simulink model "ComplexPhaseDetector"  (R2016a)
settings: Solver=VariableStepAuto  StartTime=0.0  StopTime=.01  RelTol=1e-6
InitFcn:
  | Bits = 4
  | Ts=3/280e6
  | dBRange=11
  | Br= 1/(10*Ts)
  | EbNo=50
  | FreqOffset=25000
undefined symbols (not defined in the file or in its folder): designMultirateFIR, DiscIntNeverNeededParam
libraries: xbsIndex_r4 x372, dspsigops x5, dspmlti4 x2, commchan3 x2, commdigbbndpm3 x2, simulink x2, dspfdesign x2, commrandsrc3 x2, commanabbnd3 x1
(part 1 of 5)
settings Model: Creator=frank.ziegler  LastModifiedBy=frank

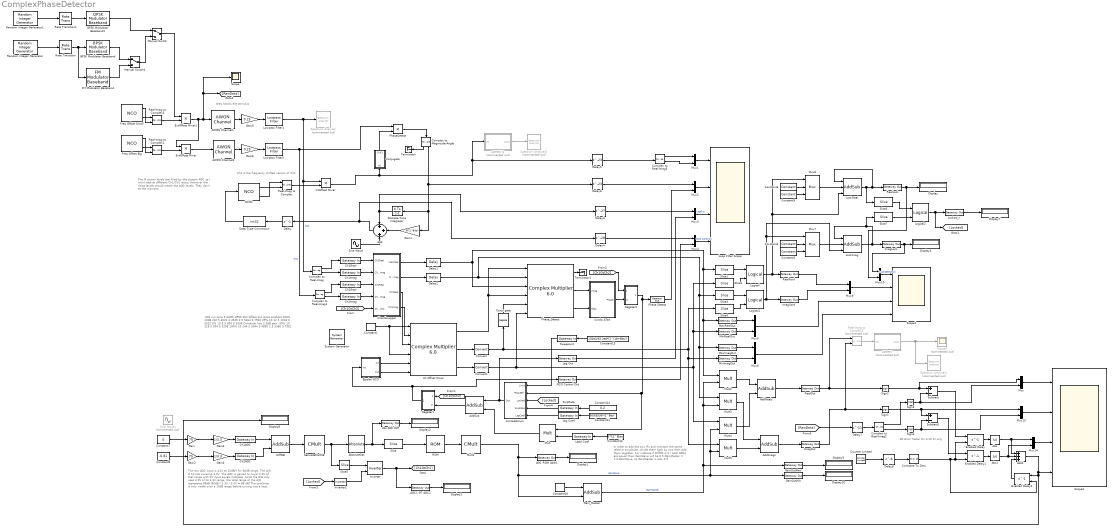
== system ComplexPhaseDetector ==
  note: Bit Error Tester for 1/10 Fs only
  note: .001 run time 9.33Mb QPSK 0Hz Offset but loops enabled
      | 100%	10dB	232
      | 		5		3022
      | 		3		4945
      | 		2.5		5464
      | 		0		7920
      |
      | 39%	10		12
      | 		5		1018
      | 		0		5332
      |
      | 0%		10		8
      | 		5		856
      | 		0		5338	Combiner has 2.5dB gain
      |
      | -39%	10		118
      | 		5		994
      | 		0		5298
      |
      | 100%	10		244
      | 		5		3044
      | 		3		4890
      | 		2.5		5386
      | 		0		7962
  note: The IF power levels are fixed by the system AGC so I won't test at different Ch1/Ch2 ratios.
      | However the noise levels should match the AGC levels. They don't at the moment.
  note: Ch2 is the frequency shifted version of Ch1.
  note: In order to add the two IFs and maintain the same relative amplitude, divide them both by two then add them together.
      | For instance if DiffDb is 0 ( both AGCs are equal) then GainSlave will be 0.5.GainMaster = 1.0-GainSlave, so GainMaster is also 0.5
  note: The raw AGC input is ±2V at 20dB/V for 80dB range.
      |
      | The A/D is 12 bits covering 3.3V. The AGC is gained to cover 3.0V of that range with 0V input equals midscale. Since the A/D only uses 3.0V of its 3.3V range, the total range of the A/D represents 88dB (80dB * 3.3V / 3.0V = 88 dB)
      |
      | The combiner is only viable over a 10dB range before turning into a best source selector. If we only use an eighth of the full range gives us 11dB.
  note: Grey blocks are stimulus
  " Freq Offset Big" : dspsigops/NCO  AccIncSrc=Specify via dialog  AccInc=floor(FreqOffset*Ts*(2^(18+Bits)))  PhaseOffsetSrc=Specify via dialog  PhaseOffset=0  AccumWL=18+Bits  HasDither=off  DitherWL=4  PNgeneratorLength=19  HasPhaseQuantizer=off  TableDepth=12  HasOutputPhaseError=off  Formula=Sine and cosine  DataType=double  OutputWL=16  OutputFL=14  CompMethod=Table lookup (no interpolation)  SampleTime=Ts  SamplesPerFrame=1  OutputFrames=off
  " Freq Offset Small" : dspsigops/NCO  AccIncSrc=Specify via dialog  AccInc=floor(FreqOffset*0.01*Ts*(2^(18+Bits)))  PhaseOffsetSrc=Specify via dialog  PhaseOffset=650000  AccumWL=18+Bits  HasDither=off  DitherWL=4  PNgeneratorLength=19  HasPhaseQuantizer=off  TableDepth=12  HasOutputPhaseError=off  Formula=Sine and cosine  DataType=double  OutputWL=16  OutputFL=14  CompMethod=Table lookup (no interpolation)  SampleTime=Ts  SamplesPerFrame=1  OutputFrames=off
  " System Generator" : xbsIndex_r4/ System Generator  Tag=genX  xilinxfamily=kintex7  part=xc7k325t  speed=-2  package=fbg676  synthesis_tool=Vivado  clock_wrapper=Clock Enables  directory=./netlist  proj_type=Vivado  Synth_file=Vivado Synthesis Defaults  Impl_file=Vivado Implementation Defaults  testbench=off  simulink_period=Ts  sysclk_period=10  dcm_input_clock_period=10  incr_netlist=off  trim_vbits=Everywhere in SubSystem  dbl_ovrd=According to Block Masks  core_generation=According to Block Masks  run_coregen=off  deprecated_control=off  eval_field=0  block_type=sysgen
  AD9957 : Subsystem  Commented=on
  AD9957-2 : Subsystem  Commented=on
  AGC ROM Addr1 : xbsIndex_r4/Gateway Out  inherit_from_input=off  hdl_port=off  rows=1  columns=1  UseAsDAC=off  DACChannel='1'  interface=None  automatic_assignment=on  address_offset=hex2dec('00')  intf_name=''  intf_description=''  timing_constraint=None  locs_specified=off  LOCs={}  io_standard={}  block_type=gatewayout
  AGC1 GT AGC2 : xbsIndex_r4/Gateway Out  inherit_from_input=off  hdl_port=on  rows=1  columns=1  UseAsDAC=off  DACChannel='1'  interface=None  automatic_assignment=on  address_offset=hex2dec('00')  intf_name=''  intf_description=''  timing_constraint=None  locs_specified=off  LOCs={}  io_standard={}  block_type=gatewayout
  AWGN Channel1 : commchan3/AWGN Channel  InputProcessing=Columns as channels (frame based)  seed=67  noiseMode="Signal to noise ratio  (Eb/No)"  EbNodB=EbNo  EsNodB=10  SNRdB=10  bitsPerSym=2  Ps=0.707  Tsym=1/Br  variance=1
  AWGN Channel2 : commchan3/AWGN Channel  InputProcessing=Columns as channels (frame based)  seed=76  noiseMode="Signal to noise ratio  (Eb/No)"  EbNodB=EbNo  EsNodB=10  SNRdB=10  bitsPerSym=2  Ps=0.707  Tsym=1/Br  variance=1
  Abs : Abs
  Abs AGC Diff : xbsIndex_r4/Gateway Out  inherit_from_input=off  hdl_port=on  rows=1  columns=1  UseAsDAC=off  DACChannel='1'  interface=None  automatic_assignment=on  address_offset=hex2dec('00')  intf_name=''  intf_description=''  timing_constraint=None  locs_specified=off  LOCs={}  io_standard={}  block_type=gatewayout
  Abs1 : Abs
  AbsoluteSat : xbsIndex_r4/Absolute  precision=User Defined  arith_type=Unsigned  n_bits=11  bin_pt=11  quantization=Truncate  overflow=Saturate  en=off  latency=1  dbl_ovrd=off  block_type=abs
  Add : Sum  Inputs=+++  OutDataTypeStr=Inherit: Same as first input
  Add1 : Sum  Inputs=+++  AccumDataTypeStr=double  OutDataTypeStr=Inherit: Same as accumulator
  AddImags : xbsIndex_r4/AddSub  mode=Addition  use_carryin=off  use_carryout=off  en=off  latency=1  precision=User Defined  arith_type="Signed  (2's comp)"  n_bits=18  bin_pt=17  quantization="Round  (unbiased: +/- Inf)"  overflow=Saturate  use_behavioral_HDL=off  hw_selection=Fabric  pipelined=off  dbl_ovrd=off  block_type=addsub
  AddReals : xbsIndex_r4/AddSub  mode=Addition  use_carryin=off  use_carryout=off  en=off  latency=1  precision=User Defined  arith_type="Signed  (2's comp)"  n_bits=18  bin_pt=17  quantization="Round  (unbiased: +/- Inf)"  overflow=Saturate  use_behavioral_HDL=off  hw_selection=Fabric  pipelined=off  dbl_ovrd=off  block_type=addsub
  AddSub : xbsIndex_r4/AddSub  mode=Addition  use_carryin=off  use_carryout=off  en=off  latency=1  precision=User Defined  arith_type="Signed  (2's comp)"  n_bits=18+Bits  bin_pt=0  quantization=Truncate  overflow=Wrap  use_behavioral_HDL=off  hw_selection=Fabric  pipelined=off  dbl_ovrd=off  block_type=addsub
  BPSK Modulator Baseband : commdigbbndpm3/BPSK Modulator Baseband  Ph=0  outDtype=double  outWordLen=16  outUDDataType=sfix(16)  outFracLenMode=Best precision  outFracLen=15  outDataTypeStr=double  outLastDataTypeStr=double
  Bipolar NCO : Subsystem
  Ch1AGC : xbsIndex_r4/Gateway In  gui_display_data_type=Fixed-point  arith_type="Signed  (2's comp)"  n_bits=12  bin_pt=11  preci_type=Single  exp_width=8  frac_width=24  rows=1  columns=1  quantization="Round  (unbiased: +/- Inf)"  overflow=Saturate  period=Ts  UseAsADC=off  ADCChannel='1'  interface=None  automatic_assignment=on  address_offset=hex2dec('00')  intf_name=''  intf_description=''  default_value=0  timing_constraint=None  locs_specified=off  LOCs={}  io_standard={}  inherit_from_input=off  hdl_port=on  dbl_ovrd=off  block_type=gatewayin
  Ch1Imag : xbsIndex_r4/Gateway In  gui_display_data_type=Fixed-point  arith_type="Signed  (2's comp)"  n_bits=18  bin_pt=17  preci_type=Single  exp_width=8  frac_width=24  rows=1  columns=1  quantization="Round  (unbiased: +/- Inf)"  overflow=Saturate  period=Ts  UseAsADC=off  ADCChannel='1'  interface=None  automatic_assignment=on  address_offset=hex2dec('00')  intf_name=''  intf_description=''  default_value=0  timing_constraint=None  locs_specified=off  LOCs={}  io_standard={}  inherit_from_input=off  hdl_port=on  dbl_ovrd=off  block_type=gatewayin
  Ch1Real : xbsIndex_r4/Gateway In  gui_display_data_type=Fixed-point  arith_type="Signed  (2's comp)"  n_bits=18  bin_pt=17  preci_type=Single  exp_width=8  frac_width=24  rows=1  columns=1  quantization="Round  (unbiased: +/- Inf)"  overflow=Saturate  period=Ts  UseAsADC=off  ADCChannel='1'  interface=None  automatic_assignment=on  address_offset=hex2dec('00')  intf_name=''  intf_description=''  default_value=0  timing_constraint=None  locs_specified=off  LOCs={}  io_standard={}  inherit_from_input=off  hdl_port=on  dbl_ovrd=off  block_type=gatewayin
  Ch2AGC : xbsIndex_r4/Gateway In  gui_display_data_type=Fixed-point  arith_type="Signed  (2's comp)"  n_bits=12  bin_pt=11  preci_type=Single  exp_width=8  frac_width=24  rows=1  columns=1  quantization="Round  (unbiased: +/- Inf)"  overflow=Saturate  period=Ts  UseAsADC=off  ADCChannel='1'  interface=None  automatic_assignment=on  address_offset=hex2dec('00')  intf_name=''  intf_description=''  default_value=0  timing_constraint=None  locs_specified=off  LOCs={}  io_standard={}  inherit_from_input=off  hdl_port=on  dbl_ovrd=off  block_type=gatewayin
  Ch2Imag : xbsIndex_r4/Gateway In  gui_display_data_type=Fixed-point  arith_type="Signed  (2's comp)"  n_bits=18  bin_pt=17  preci_type=Single  exp_width=8  frac_width=24  rows=1  columns=1  quantization="Round  (unbiased: +/- Inf)"  overflow=Saturate  period=Ts  UseAsADC=off  ADCChannel='1'  interface=None  automatic_assignment=on  address_offset=hex2dec('00')  intf_name=''  intf_description=''  default_value=0  timing_constraint=None  locs_specified=off  LOCs={}  io_standard={}  inherit_from_input=off  hdl_port=on  dbl_ovrd=off  block_type=gatewayin
  Ch2Real : xbsIndex_r4/Gateway In  gui_display_data_type=Fixed-point  arith_type="Signed  (2's comp)"  n_bits=18  bin_pt=17  preci_type=Single  exp_width=8  frac_width=24  rows=1  columns=1  quantization="Round  (unbiased: +/- Inf)"  overflow=Saturate  period=Ts  UseAsADC=off  ADCChannel='1'  interface=None  automatic_assignment=on  address_offset=hex2dec('00')  intf_name=''  intf_description=''  default_value=0  timing_constraint=None  locs_specified=off  LOCs={}  io_standard={}  inherit_from_input=off  hdl_port=on  dbl_ovrd=off  block_type=gatewayin
  ChanSwapper : Subsystem
  Compare To Zero : simulink/Logic and Bit Operations/Compare To Zero  relop===  OutDataTypeStr=boolean
  Complex to Magnitude-Angle : ComplexToMagnitudeAngle
  Complex to Real-Imag{,1..2,5} (4 alike) : ComplexToRealImag
  Conju gate : xbsIndex_r4/Negate  precision=User Defined  arith_type="Signed  (2's comp)"  n_bits=18  bin_pt=17  quantization=Truncate  overflow=Saturate  en=off  latency=0  dbl_ovrd=off  block_type=negate
  Conjugate : Subsystem
  Constant1 : xbsIndex_r4/Constant  const=1  gui_display_data_type=Boolean  arith_type=Boolean  n_bits=16  bin_pt=14  preci_type=Single  exp_width=8  frac_width=24  explicit_period=on  period=Ts  equ=P=C  opselect=C  inp2=PCIN>>17  opr=+  inp1=P  carry=CIN  dbl_ovrd=off  block_type=constant
  Constant10 : xbsIndex_r4/Constant  const=1.0  gui_display_data_type=Fixed-point  arith_type=Unsigned  n_bits=18  bin_pt=18  preci_type=Single  exp_width=8  frac_width=24  explicit_period=on  period=Ts  equ=P=C  opselect=C  inp2=PCIN>>17  opr=+  inp1=P  carry=CIN  dbl_ovrd=off  block_type=constant
  Constant11 : Constant  Value=50/65536*(2^Bits)  OutDataTypeStr=double
  Constant12 : Constant  Value=5*(2^Bits)  OutDataTypeStr=double
  Constant13 : Constant  Value=130e3/93.3e6*(2^(18+Bits))  OutDataTypeStr=double
  Constant14 : Constant  Value=0.2  OutDataTypeStr=double
  Constant4 : xbsIndex_r4/Constant  const=1  gui_display_data_type=Fixed-point  arith_type=Unsigned  n_bits=8  bin_pt=0  preci_type=Single  exp_width=8  frac_width=24  explicit_period=off  period=1  equ=P=C  opselect=C  inp2=PCIN>>17  opr=+  inp1=P  carry=CIN  dbl_ovrd=off  block_type=constant
  Constant5 : xbsIndex_r4/Constant  const=2  gui_display_data_type=Fixed-point  arith_type=Unsigned  n_bits=8  bin_pt=0  preci_type=Single  exp_width=8  frac_width=24  explicit_period=off  period=1  equ=P=C  opselect=C  inp2=PCIN>>17  opr=+  inp1=P  carry=CIN  dbl_ovrd=off  block_type=constant
  Constant6 : xbsIndex_r4/Constant  const=1  gui_display_data_type=Fixed-point  arith_type=Unsigned  n_bits=8  bin_pt=0  preci_type=Single  exp_width=8  frac_width=24  explicit_period=off  period=1  equ=P=C  opselect=C  inp2=PCIN>>17  opr=+  inp1=P  carry=CIN  dbl_ovrd=off  block_type=constant
  Constant7 : Constant  Value=0  OutDataTypeStr=double
  Constant8 : Constant  Value=-0.81  OutDataTypeStr=double
  Constant9 : xbsIndex_r4/Constant  const=2  gui_display_data_type=Fixed-point  arith_type=Unsigned  n_bits=8  bin_pt=0  preci_type=Single  exp_width=8  frac_width=24  explicit_period=off  period=1  equ=P=C  opselect=C  inp2=PCIN>>17  opr=+  inp1=P  carry=CIN  dbl_ovrd=off  block_type=constant
  Convert : xbsIndex_r4/Convert  gui_display_data_type=Fixed-point  arith_type="Signed  (2's comp)"  n_bits=18  bin_pt=17  float_type=Single  exp_bits=8  fraction_bits=24  quantization=Truncate  overflow=Saturate  en=off  latency=1  pipeline=off  dbl_ovrd=off  block_type=convert
  Convert1 : xbsIndex_r4/Convert  gui_display_data_type=Fixed-point  arith_type="Signed  (2's comp)"  n_bits=18  bin_pt=17  float_type=Single  exp_bits=8  fraction_bits=24  quantization=Truncate  overflow=Saturate  en=off  latency=1  pipeline=off  dbl_ovrd=off  block_type=convert
  Cordic ATan : Subsystem
  Counter Limited : simulink/Sources/Counter Limited  uplimit=9  tsamp=-1
  Data Type Conversion : DataTypeConversion  OutDataTypeStr=int32  SaturateOnIntegerOverflow=on
  Delay : Delay  DelayLength=1
  Delay1 : xbsIndex_r4/Delay  rst=off  infoeditControl=Selection of Reset will increase slice count due to use of real FFs and instead of SRLs  en=off  latency=4  reg_retiming=off  dbl_ovrd=off  block_type=delay
  Delay2 : xbsIndex_r4/Delay  rst=off  infoeditControl=Selection of Reset will increase slice count due to use of real FFs and instead of SRLs  en=off  latency=4  reg_retiming=off  dbl_ovrd=off  block_type=delay
  Delay3 : Delay  DelayLength=27
  Delay4 : Delay  DelayLength=28
  Delay5 : Delay  DelayLength=23
  Delay6 : Delay  DelayLength=23
  Delay7 : Delay  DelayLength=11
  Delay8 : Delay  DelayLength=6
  DiffDB : xbsIndex_r4/AddSub  mode=Subtraction  use_carryin=off  use_carryout=off  en=off  latency=1  precision=User Defined  arith_type="Signed  (2's comp)"  n_bits=12  bin_pt=11  quantization=Truncate  overflow=Saturate  use_behavioral_HDL=off  hw_selection=Fabric  pipelined=off  dbl_ovrd=off  block_type=addsub
  Discrete-Time Integrator : DiscreteIntegrator  gainval=(2^Bits)*50/65536/Ts  InitialConditionSetting=State (most efficient)  SampleTime=Ts  ICPrevOutput=DiscIntNeverNeededParam  ICPrevScaledInput=DiscIntNeverNeededParam
  Display{,1..4,7..10} (9 alike) : Display
  Enabled Delay : Delay  DelayLength=1  ShowEnablePort=on
      settings: InputPortMap=u0,e6
  Enabled Delay1 : Delay  DelayLength=1  ShowEnablePort=on
      settings: InputPortMap=u0,e6
  Enabled Delay2 : Delay  DelayLength=1  ShowEnablePort=on
      settings: InputPortMap=u0,e6
  ExtOffset Mixer : Product
  ExtOffset Mixer1 : Product
  FM Modulator Baseband : commanabbnd3/FM Modulator Baseband  FrequencyDeviation=100000  SimulateUsing=Code generation
  Gain : Gain  Gain=.75
  Gain1 : Gain  Gain=5*(2^Bits)
  Gain2 : Gain  Gain=.75
  Gain3 : Gain  Gain=1/3.3
  Gain4 : Gain  Gain=1/3.3
  Gain5 : Gain  Gain=0.25
  Gain6 : Gain  Gain=0.25
  GainOutMax : xbsIndex_r4/Gateway Out  inherit_from_input=off  hdl_port=on  rows=1  columns=1  UseAsDAC=off  DACChannel='1'  interface=None  automatic_assignment=on  address_offset=hex2dec('00')  intf_name=''  intf_description=''  timing_constraint=None  locs_specified=off  LOCs={}  io_standard={}  block_type=gatewayout
  GainOutMin : xbsIndex_r4/Gateway Out  inherit_from_input=off  hdl_port=on  rows=1  columns=1  UseAsDAC=off  DACChannel='1'  interface=None  automatic_assignment=on  address_offset=hex2dec('00')  intf_name=''  intf_description=''  timing_constraint=None  locs_specified=off  LOCs={}  io_standard={}  block_type=gatewayout
  Gain_Master : xbsIndex_r4/AddSub  mode=Subtraction  use_carryin=off  use_carryout=off  en=off  latency=0  precision=User Defined  arith_type=Unsigned  n_bits=18  bin_pt=18  quantization=Truncate  overflow=Wrap  use_behavioral_HDL=off  hw_selection=Fabric  pipelined=off  dbl_ovrd=off  block_type=addsub
  ImagLock : xbsIndex_r4/Gateway Out  inherit_from_input=off  hdl_port=on  rows=1  columns=1  UseAsDAC=off  DACChannel='1'  interface=None  automatic_assignment=on  address_offset=hex2dec('00')  intf_name=''  intf_description=''  timing_constraint=None  locs_specified=off  LOCs={}  io_standard={}  block_type=gatewayout
  ImagOut : xbsIndex_r4/Gateway Out  inherit_from_input=off  hdl_port=on  rows=1  columns=1  UseAsDAC=off  DACChannel='1'  interface=None  automatic_assignment=on  address_offset=hex2dec('00')  intf_name=''  intf_description=''  timing_constraint=None  locs_specified=off  LOCs={}  io_standard={}  block_type=gatewayout
  ImagXord : xbsIndex_r4/Gateway Out  inherit_from_input=off  hdl_port=on  rows=1  columns=1  UseAsDAC=off  DACChannel='1'  interface=None  automatic_assignment=on  address_offset=hex2dec('00')  intf_name=''  intf_description=''  timing_constraint=None  locs_specified=off  LOCs={}  io_standard={}  block_type=gatewayout
  Int Offset Mixer : xbsIndex_r4/Complex Multiplier 6.0   hasatlast=off  hasatuser=off  atuserwidth=1  hasbtlast=off  hasbtuser=off  btuserwidth=1  multtype=Use_Mults  optimizegoal=Resources  flowcontrol=NonBlocking  outputwidth=20  roundmode=Truncate  hasctrltlast=off  hasctrltuser=off  ctrltuserwidth=1  outtlastbehv=Null  latencyconfig=Manual  minimumlatency=3  aclken=off  aresetn=off  trim_axipin_name=on  simulation_type=hybrid_sim  simulation_model=sysgen:cmpy_v6_0  data_path_portlist={ 's_axis_a_tdata_real', 's_axis_a_tdata_imag', 's_axis_b_tdata_real', 's_axis_b_tdata_imag', 's_axis_ctrl_tdata_rounding_bit', 'm_axis_dout_tdata_real', 'm_axis_dout_tdata_imag' }  aportwidth=63  bportwidth=63  ip_name=Complex Multiplier  ip_version=6.0  dsptool_ready=true  ipcore_usecache=true  ipcore_useipmodelcache=true  ipcore_verbose=false  ipcore_latency_parameter='minimumlatency'  wrapper_available=true  port_translation_map={ 'aclken' => 'en', 'aresetn' => 'rst'}  block_type=cmpy_v6_0
  IntOffset Mixer : Product
  Inverter : xbsIndex_r4/Inverter  en=on  latency=01  dbl_ovrd=off  block_type=inv
  Inverter2 : xbsIndex_r4/Inverter  en=off  latency=0  dbl_ovrd=off  block_type=inv
  Lag Coef : xbsIndex_r4/Gateway In  gui_display_data_type=Fixed-point  arith_type="Signed  (2's comp)"  n_bits=18  bin_pt=17  preci_type=Single  exp_width=8  frac_width=24  rows=1  columns=1  quantization="Round  (unbiased: +/- Inf)"  overflow=Wrap  period=Ts  UseAsADC=off  ADCChannel='1'  interface=None  automatic_assignment=on  address_offset=hex2dec('00')  intf_name='axi4'  intf_description='Lead Coefficient'  default_value=5*Ts  timing_constraint=None  locs_specified=off  LOCs={}  io_standard={}  inherit_from_input=off  hdl_port=on  dbl_ovrd=off  block_type=gatewayin
  Lag Out : xbsIndex_r4/Gateway Out  inherit_from_input=off  hdl_port=on  rows=1  columns=1  UseAsDAC=off  DACChannel='1'  interface=None  automatic_assignment=on  address_offset=hex2dec('00')  intf_name=''  intf_description=''  timing_constraint=None  locs_specified=off  LOCs={}  io_standard={}  block_type=gatewayout
  Lead Coef : xbsIndex_r4/Gateway In  gui_display_data_type=Fixed-point  arith_type="Signed  (2's comp)"  n_bits=18  bin_pt=9  preci_type=Single  exp_width=8  frac_width=24  rows=1  columns=1  quantization="Round  (unbiased: +/- Inf)"  overflow=Wrap  period=Ts  UseAsADC=off  ADCChannel='1'  interface=None  automatic_assignment=on  address_offset=hex2dec('00')  intf_name='axi4'  intf_description='Lead Coefficient'  default_value=10  timing_constraint=None  locs_specified=off  LOCs={}  io_standard={}  inherit_from_input=off  hdl_port=on  dbl_ovrd=off  block_type=gatewayin
  LimitedAccum : Subsystem
  LockImag : xbsIndex_r4/AddSub  mode=Addition or Subtraction  use_carryin=off  use_carryout=off  en=off  latency=1  precision=User Defined  arith_type=Unsigned  n_bits=13  bin_pt=0  quantization=Truncate  overflow=Saturate  use_behavioral_HDL=off  hw_selection=Fabric  pipelined=off  dbl_ovrd=off  block_type=addsub
  LockReal : xbsIndex_r4/AddSub  mode=Addition or Subtraction  use_carryin=off  use_carryout=off  en=off  latency=1  precision=User Defined  arith_type=Unsigned  n_bits=13  bin_pt=0  quantization=Truncate  overflow=Saturate  use_behavioral_HDL=off  hw_selection=Fabric  pipelined=off  dbl_ovrd=off  block_type=addsub
  Locked_n : xbsIndex_r4/Gateway Out  inherit_from_input=off  hdl_port=on  rows=1  columns=1  UseAsDAC=off  DACChannel='1'  interface=None  automatic_assignment=on  address_offset=hex2dec('00')  intf_name=''  intf_description=''  timing_constraint=None  locs_specified=off  LOCs={}  io_standard={}  block_type=gatewayout
  Logical : xbsIndex_r4/Logical  logical_function=XOR  inputs=2  en=off  latency=1  precision=Full  arith_type=Unsigned  n_bits=16  bin_pt=0  align_bp=on  dbl_ovrd=off  block_type=logical
  Logical1 : xbsIndex_r4/Logical  logical_function=XOR  inputs=2  en=off  latency=1  precision=Full  arith_type=Unsigned  n_bits=16  bin_pt=0  align_bp=on  dbl_ovrd=off  block_type=logical
  Logical2 : xbsIndex_r4/Logical  logical_function=OR  inputs=2  en=off  latency=1  precision=Full  arith_type=Unsigned  n_bits=16  bin_pt=0  align_bp=on  dbl_ovrd=off  block_type=logical
  Loop Filter Scope : Scope  NumInputPorts=4
  Lowpass Filter1 : dspfdesign/Lowpass Filter  FilterType=FIR  DesignForMinimumOrder=on  FilterOrder=50  PassbandFrequency=Br/2  StopbandFrequency=46e6  PassbandRipple=0.1  StopbandAttenuation=80  InheritSampleRate=off  SampleRate=1/Ts  roundingMode=Floor  coeffsDataTypeStr=fixdt(1,16)  SimulateUsing=Interpreted execution
  Lowpass Filter2 : dspfdesign/Lowpass Filter  FilterType=FIR  DesignForMinimumOrder=on  FilterOrder=50  PassbandFrequency=Br/2  StopbandFrequency=46e6  PassbandRipple=0.1  StopbandAttenuation=80  InheritSampleRate=off  SampleRate=1/Ts  roundingMode=Floor  coeffsDataTypeStr=fixdt(1,16)  SimulateUsing=Interpreted execution
  Manual Switch : ManualSwitch
  Manual Switch1 : ManualSwitch
  MaxImagOut : xbsIndex_r4/Gateway Out  inherit_from_input=off  hdl_port=on  rows=1  columns=1  UseAsDAC=off  DACChannel='1'  interface=None  automatic_assignment=on  address_offset=hex2dec('00')  intf_name=''  intf_description=''  timing_constraint=None  locs_specified=off  LOCs={}  io_standard={}  block_type=gatewayout
  MaxRealOut : xbsIndex_r4/Gateway Out  inherit_from_input=off  hdl_port=on  rows=1  columns=1  UseAsDAC=off  DACChannel='1'  interface=None  automatic_assignment=on  address_offset=hex2dec('00')  intf_name=''  intf_description=''  timing_constraint=None  locs_specified=off  LOCs={}  io_standard={}  block_type=gatewayout
  MinImagOut : xbsIndex_r4/Gateway Out  inherit_from_input=off  hdl_port=on  rows=1  columns=1  UseAsDAC=off  DACChannel='1'  interface=None  automatic_assignment=on  address_offset=hex2dec('00')  intf_name=''  intf_description=''  timing_constraint=None  locs_specified=off  LOCs={}  io_standard={}  block_type=gatewayout
  MinRealOut : xbsIndex_r4/Gateway Out  inherit_from_input=off  hdl_port=on  rows=1  columns=1  UseAsDAC=off  DACChannel='1'  interface=None  automatic_assignment=on  address_offset=hex2dec('00')  intf_name=''  intf_description=''  timing_constraint=None  locs_specified=off  LOCs={}  io_standard={}  block_type=gatewayout
  Mult : xbsIndex_r4/Mult  precision=User Defined  arith_type="Signed  (2's comp)"  n_bits=18+Bits  bin_pt=9  quantization="Round  (unbiased: +/- Inf)"  overflow=Wrap  en=off  latency=4  use_behavioral_HDL=off  opt=Speed  use_embedded=on  optimum_pipeline=off  pipeline=on  dbl_ovrd=off  use_rpm=on  placement_style=Triangular  block_type=mult
  Mult1 : xbsIndex_r4/CMult  const=0.5  gui_display_data_type=Fixed-point  const_n_bits=4  const_bin_pt=3  float_type=Single  exp_bits=8  fraction_bits=24  en=off  latency=0  precision=User Defined  arith_type=Unsigned  n_bits=18  bin_pt=18  quantization=Truncate  overflow=Wrap  use_behavioral_HDL=off  mem_type=Distributed RAM  pipeline=off  dbl_ovrd=off  block_type=cmult
  Mult{2..5} (4 alike) : xbsIndex_r4/Mult  precision=User Defined  arith_type="Signed  (2's comp)"  n_bits=18  bin_pt=17  quantization="Round  (unbiased: +/- Inf)"  overflow=Wrap  en=off  latency=3  use_behavioral_HDL=off  opt=Speed  use_embedded=on  optimum_pipeline=off  pipeline=on  dbl_ovrd=off  use_rpm=on  placement_style=Triangular  block_type=mult
  Mux{,1..6,9..10,13..14} (11 alike) : Mux  Inputs=2
  Mux7 : xbsIndex_r4/Mux  inputs=2  en=off  latency=0  precision=Full  arith_type=Unsigned  n_bits=16  bin_pt=14  quantization=Truncate  overflow=Wrap  dbl_ovrd=off  block_type=mux
  Mux8 : xbsIndex_r4/Mux  inputs=2  en=off  latency=0  precision=Full  arith_type=Unsigned  n_bits=16  bin_pt=14  quantization=Truncate  overflow=Wrap  dbl_ovrd=off  block_type=mux
  NCO Control Out : xbsIndex_r4/Gateway Out  inherit_from_input=off  hdl_port=on  rows=1  columns=1  UseAsDAC=off  DACChannel='1'  interface=None  automatic_assignment=on  address_offset=hex2dec('00')  intf_name=''  intf_description=''  timing_constraint=None  locs_specified=off  LOCs={}  io_standard={}  block_type=gatewayout
  NCO1 : dspsigops/NCO  AccIncSrc=Input port  AccInc=100  PhaseOffsetSrc=Specify via dialog  PhaseOffset=0  AccumWL=18+Bits  HasDither=off  DitherWL=4  PNgeneratorLength=19  HasPhaseQuantizer=off  TableDepth=12  HasOutputPhaseError=off  Formula=Sine and cosine  DataType=double  OutputWL=16  OutputFL=14  CompMethod=Table lookup (no interpolation)  SampleTime=Ts  SamplesPerFrame=1  OutputFrames=off
  Negater1 : Subsystem
  Negater2 : Subsystem
  Phase Detect : xbsIndex_r4/Gateway Out  inherit_from_input=off  hdl_port=on  rows=1  columns=1  UseAsDAC=off  DACChannel='1'  interface=None  automatic_assignment=on  address_offset=hex2dec('00')  intf_name=''  intf_description=''  timing_constraint=None  locs_specified=off  LOCs={}  io_standard={}  block_type=gatewayout
  PhaseDetect : Product
  Phase_Detect : xbsIndex_r4/Complex Multiplier 6.0   hasatlast=off  hasatuser=off  atuserwidth=1  hasbtlast=off  hasbtuser=off  btuserwidth=1  multtype=Use_Mults  optimizegoal=Resources  flowcontrol=NonBlocking  outputwidth=18  roundmode=Truncate  hasctrltlast=off  hasctrltuser=off  ctrltuserwidth=1  outtlastbehv=Null  latencyconfig=Automatic  minimumlatency=37  aclken=off  aresetn=off  trim_axipin_name=on  simulation_type=hybrid_sim  simulation_model=sysgen:cmpy_v6_0  data_path_portlist={ 's_axis_a_tdata_real', 's_axis_a_tdata_imag', 's_axis_b_tdata_real', 's_axis_b_tdata_imag', 's_axis_ctrl_tdata_rounding_bit', 'm_axis_dout_tdata_real', 'm_axis_dout_tdata_imag' }  aportwidth=63  bportwidth=63  ip_name=Complex Multiplier  ip_version=6.0  dsptool_ready=true  ipcore_usecache=true  ipcore_useipmodelcache=true  ipcore_verbose=false  ipcore_latency_parameter='minimumlatency'  wrapper_available=true  port_translation_map={ 'aclken' => 'en', 'aresetn' => 'rst'}  block_type=cmpy_v6_0
  QPSK Modulator Baseband1 : commdigbbndpm3/QPSK Modulator Baseband  InType=Integer  Enc=Gray  Ph=pi/4  outDtype=double  outWordLen=16  outUDDataType=sfix(16)  outFracLenMode=Best precision  outFracLen=15  outDataTypeStr=double  outLastDataTypeStr=double
  ROM : xbsIndex_r4/ROM  depth=1024  initVector=[10.^((0:1022)*(-(dBRange/20))/1023) 0]  distributed_mem=Block RAM  rst=off  init_reg=0  en=off  latency=1  gui_display_data_type=Fixed-point  arith_type=Unsigned  n_bits=18  bin_pt=18  preci_type=Single  exp_width=8  frac_width=24  optimize=Area  use_rpm=on  dbl_ovrd=off  block_type=sprom
  Random Integer Generator : commrandsrc3/Random Integer Generator  SetSize=2  SeedSource=Auto  Seed=0  SampleTime=1/Br  SamplesPerFrame=1  OutputDataType=double  SimulateUsing=Code generation
  Random Integer Generator1 : commrandsrc3/Random Integer Generator  SetSize=4  SeedSource=Auto  Seed=0  SampleTime=1/Br  SamplesPerFrame=1  OutputDataType=double  SimulateUsing=Code generation
  Rate Transition : RateTransition  OutPortSampleTime=Ts
  Rate Transition1 : RateTransition  OutPortSampleTime=Ts
  Real-Imag to Complex : RealImagToComplex
  Real-Imag to Complex1 : RealImagToComplex
  Real-Imag to Complex2 : RealImagToComplex  Commented=on
  Real-Imag to Complex3 : RealImagToComplex
  RealLock : xbsIndex_r4/Gateway Out  inherit_from_input=off  hdl_port=on  rows=1  columns=1  UseAsDAC=off  DACChannel='1'  interface=None  automatic_assignment=on  address_offset=hex2dec('00')  intf_name=''  intf_description=''  timing_constraint=None  locs_specified=off  LOCs={}  io_standard={}  block_type=gatewayout
  RealOut : xbsIndex_r4/Gateway Out  inherit_from_input=off  hdl_port=on  rows=1  columns=1  UseAsDAC=off  DACChannel='1'  interface=None  automatic_assignment=on  address_offset=hex2dec('00')  intf_name=''  intf_description=''  timing_constraint=None  locs_specified=off  LOCs={}  io_standard={}  block_type=gatewayout
  RealXord : xbsIndex_r4/Gateway Out  inherit_from_input=off  hdl_port=on  rows=1  columns=1  UseAsDAC=off  DACChannel='1'  interface=None  automatic_assignment=on  address_offset=hex2dec('00')  intf_name=''  intf_description=''  timing_constraint=None  locs_specified=off  LOCs={}  io_standard={}  block_type=gatewayout
  SaturateMultX8 : xbsIndex_r4/CMult  const=8  gui_display_data_type=Fixed-point  const_n_bits=4  const_bin_pt=0  float_type=Single  exp_bits=8  fraction_bits=24  en=off  latency=0  precision=User Defined  arith_type="Signed  (2's comp)"  n_bits=18  bin_pt=17  quantization=Truncate  overflow=Saturate  use_behavioral_HDL=off  mem_type=Distributed RAM  pipeline=off  dbl_ovrd=off  block_type=cmult
  Scope : Scope
  Scope1 : Scope  NumInputPorts=4
  Scope3 : Scope  NumInputPorts=4
  Scope5 : Scope  Commented=on
  Sign{1..4} (4 alike) : Signum
  Sine Wave : Sin  Amplitude=0  Frequency=2*2*pi()  SampleTime=Ts
  Sine Wave1 : Sin  Commented=on  Frequency=2000  SampleTime=Ts
  Slice : xbsIndex_r4/Slice  nbits=10  boolean_output=off  mode=Upper Bit Location + Width  bit1=0  base1=MSB of Input  bit0=0  base0=LSB of Input  dbl_ovrd=off  block_type=slice
  Slice{1..7} (7 alike) : xbsIndex_r4/Slice  nbits=1  boolean_output=on  mode=Upper Bit Location + Width  bit1=0  base1=MSB of Input  bit0=0  base0=LSB of Input  dbl_ovrd=off  block_type=slice
  Spectrum Analyzer : SpectrumAnalyzer  Commented=on
  Spectrum Analyzer1 : SpectrumAnalyzer  Commented=on
  Spectrum Analyzer2 : SpectrumAnalyzer  Commented=on
  Subtract : Sum  Inputs=+-
  Subtract1 : Sum  Inputs=+-
  SweepLmt : xbsIndex_r4/Gateway In  gui_display_data_type=Fixed-point  arith_type="Signed  (2's comp)"  n_bits=10+Bits  bin_pt=0  preci_type=Single  exp_width=8  frac_width=24  rows=1  columns=1  quantization="Round  (unbiased: +/- Inf)"  overflow=Wrap  period=Ts  UseAsADC=off  ADCChannel='1'  interface=None  automatic_assignment=on  address_offset=hex2dec('00')  intf_name='axi4'  intf_description='Lead Coefficient'  default_value=5*Ts  timing_constraint=None  locs_specified=off  LOCs={}  io_standard={}  inherit_from_input=off  hdl_port=on  dbl_ovrd=off  block_type=gatewayin
  SwpRate : xbsIndex_r4/Gateway In  gui_display_data_type=Fixed-point  arith_type="Signed  (2's comp)"  n_bits=18  bin_pt=9  preci_type=Single  exp_width=8  frac_width=24  rows=1  columns=1  quantization="Round  (unbiased: +/- Inf)"  overflow=Wrap  period=Ts  UseAsADC=off  ADCChannel='1'  interface=None  automatic_assignment=on  address_offset=hex2dec('00')  intf_name='axi4'  intf_description='Lead Coefficient'  default_value=5*Ts  timing_constraint=None  locs_specified=off  LOCs={}  io_standard={}  inherit_from_input=off  hdl_port=on  dbl_ovrd=off  block_type=gatewayin
  Terminator : Terminator
  Terminator1 : Terminator
  wires:
  Real-Imag to Complex/1 -> IntOffset Mixer/2
  PhaseDetect/1 -> Complex to Magnitude-Angle/1
  Conjugate/1(Out1) -> PhaseDetect/2
  NCO1/2 -> Real-Imag to Complex/1
  NCO1/1 -> Real-Imag to Complex/2
  Discrete-Time Integrator/1 -> Delay3/1, Add/1
  Gain1/1 -> Add/2
  Sine Wave/1 -> Add/3
  ExtOffset Mixer1/1 -> ExtOffset Mixer/1, Scope/1, [RawData], AWGN Channel1/1
  " Freq Offset Big"/1 -> Real-Imag to Complex1/2
  " Freq Offset Big"/2 -> Real-Imag to Complex1/1
  Real-Imag to Complex1/1 -> ExtOffset Mixer/2
  IntOffset Mixer/1 -> AD9957-2/1(In1), Delay5/1, Conjugate/1(In1)
  Complex to Magnitude-Angle/2 -> Delay6/1, Gain1/1, Discrete-Time Integrator/1
  Complex to Real-Imag/1 -> Ch1Real/1
  Complex to Real-Imag/2 -> Ch1Imag/1
  Complex to Real-Imag1/2 -> Ch2Imag/1
  Complex to Real-Imag1/1 -> Ch2Real/1
  Int Offset Mixer/2 -> Convert/1
  Int Offset Mixer/1 -> Phase_Detect/4, Phase_Detect/1
  Conju gate/1 -> Phase_Detect/5
  Complex to Magnitude-Angle/1 -> Terminator/1
  Constant1/1 -> Int Offset Mixer/4, Int Offset Mixer/1
  Mult/1 -> AddSub/2
  Phase Detect/1 -> Mux2/2
  Int Offset Mixer/3 -> Convert1/1
  Lead Coef/1 -> Mult/2
  Lag Coef/1 -> LimitedAccum/5(LagCoef)
  Data Type Conversion/1 -> NCO1/1
  Bipolar NCO/1(sin) -> Int Offset Mixer/5
  Bipolar NCO/2(cos) -> Int Offset Mixer/6
  Phase_Detect/1 -> Terminator1/1
  MaxRealOut/1 -> Mux5/1
  MaxImagOut/1 -> Mux6/1
  MinImagOut/1 -> Mux6/2
  MinRealOut/1 -> Mux5/2
  Convert/1 -> MinImagOut/1, Mult5/1, Slice4/1, Conju gate/1
  Convert1/1 -> Phase_Detect/6, Slice2/1, MinRealOut/1, Mult4/1
  Mux5/1 -> Scope1/3
  Mux6/1 -> Scope1/4
  Mult1/1 -> AGC ROM Addr1/1, Gain_Master/2, GainOutMin/1, Mult4/2, Mult5/2  "GainSlave"
  Ch1AGC/1 -> DiffDB/1
  Ch2AGC/1 -> DiffDB/2
  DiffDB/1 -> SaturateMultX8/1
  Constant8/1 -> Gain2/1
  Gain/1 -> Gain3/1
  Gain2/1 -> Gain4/1
  Gain4/1 -> Ch2AGC/1
  Gain3/1 -> Ch1AGC/1
  AbsoluteSat/1 -> Slice/1, Abs AGC Diff/1
  Abs AGC Diff/1 -> Display2/1
  AGC1 GT AGC2/1 -> Display3/1
  SaturateMultX8/1 -> AbsoluteSat/1, Slice5/1
  Mult2/1 -> AddReals/1
  Mult4/1 -> AddReals/2
  Mult5/1 -> AddImags/2
  Mult3/1 -> AddImags/1
  AddReals/1 -> RealOut/1
  Inverter/1 -> [Ch1GtCh2], AGC1 GT AGC2/1
  Constant10/1 -> Gain_Master/1
  ROM/1 -> Mult1/1
  RealOut/1 -> Sign2/1, Real-Imag to Complex2/1
  ImagOut/1 -> Real-Imag to Complex2/2, Sign1/1
  AddImags/1 -> ImagOut/1
  Constant11/1 -> Lag Coef/1
  Constant12/1 -> Lead Coef/1
  AWGN Channel1/1 -> Gain5/1
  Gain5/1 -> Lowpass Filter1/1
  Phase_Detect/2 -> Cordic ATan/1(Imag)
  Phase_Detect/3 -> Cordic ATan/2(Real)
  AWGN Channel2/1 -> Gain6/1
  Gain6/1 -> Lowpass Filter2/1
  ExtOffset Mixer/1 -> AWGN Channel2/1
  Complex to Real-Imag5/1 -> Mux1/1
  Complex to Real-Imag5/2 -> Mux1/2
  Lag Out/1 -> Mux3/2
  Real-Imag to Complex2/1 -> AD9957/1(In1)
  Rate Transition/1 -> FM Modulator Baseband/1, BPSK Modulator Baseband/1
  Random Integer Generator/1 -> Rate Transition/1
  AD9957/1(Out1) -> Scope5/1, Spectrum Analyzer1/1
  Delay3/1 -> Mux3/1
  Delay5/1 -> Complex to Real-Imag5/1
  Delay6/1 -> Mux2/1
  AD9957-2/1(Out1) -> Spectrum Analyzer2/1
  Slice/1 -> ROM/1
  AGC ROM Addr1/1 -> Display1/1
  Slice1/1 -> Logical/1
  Slice2/1 -> Logical/2
  RealXord/1 -> Mux9/1
  Slice3/1 -> Logical1/1
  Slice4/1 -> Logical1/2
  ImagXord/1 -> Mux9/2
  LockReal/1 -> Slice6/1, LockReal/1, RealLock/1
  RealLock/1 -> Mux10/2, Display/1
  Mux9/1 -> Scope1/2
  Logical1/1 -> LockImag/3, Mux7/1, ImagXord/1
  LockImag/1 -> Slice7/1, LockImag/1, ImagLock/1
  Mux7/1 -> LockImag/2
  ImagLock/1 -> Display4/1, Mux10/1
  Mux10/1 -> Scope1/1  "LockDetectors"
  [Ch1GtCh2] -> ChanSwapper/5(Ch1GtCh2)
  Slice5/1 -> Inverter/1
  Delay/1 -> Data Type Conversion/1
  Mux3/1 -> Loop Filter Scope/3  "LagOut"
  Mux4/1 -> Loop Filter Scope/4  "NCO Controls"
  Delay4/1 -> Mux4/1
  NCO Control Out/1 -> Mux4/2
  Ch1Imag/1 -> ChanSwapper/2(Ch1Imag)
  Ch2Real/1 -> ChanSwapper/3(Ch2Real)
  Ch2Imag/1 -> ChanSwapper/4(Ch2Imag)
  Ch1Real/1 -> ChanSwapper/1(Ch1Real)
  ChanSwapper/4(MinImag) -> Int Offset Mixer/2
  ChanSwapper/3("MinReal ") -> Int Offset Mixer/3
  Lowpass Filter1/1 -> Spectrum Analyzer/1, Complex to Real-Imag/1, IntOffset Mixer/1  "Ch1"
  Lowpass Filter2/1 -> PhaseDetect/1, Complex to Real-Imag1/1  "Ch2"
  Constant4/1 -> Mux7/2
  Constant5/1 -> Mux7/3
  Logical/1 -> Mux8/1, LockReal/3, RealXord/1
  Mux8/1 -> LockReal/2
  Constant6/1 -> Mux8/2
  Constant9/1 -> Mux8/3
  Negater1/1(Out) -> NCO Control Out/1, Bipolar NCO/1(Inc)
  [Ch1GtCh2] -> Negater1/1(Sel)
  AddSub/1 -> Negater1/2(In)
  Cordic ATan/1(Phase) -> Negater2/2(In)
  [Ch1GtCh2] -> Negater2/1(Sel)
  Add/1 -> Delay4/1, Delay/1
  Slice7/1 -> Logical2/2
  Slice6/1 -> Logical2/1
  Logical2/1 -> Locked_n/1, [Locked]
  Locked_n/1 -> Display7/1
  Mux1/1 -> Loop Filter Scope/1
  Mux2/1 -> Loop Filter Scope/2
  [Locked] -> Inverter2/1
  LimitedAccum/1(Out) -> AddSub/1, Lag Out/1
  Negater2/1(Out) -> LimitedAccum/2(PhaseErr), Mult/1, Phase Detect/1
  SweepLmt/1 -> LimitedAccum/1(Limit)
  Constant13/1 -> SweepLmt/1
  ChanSwapper/1(MaxReal) -> Delay1/1
  ChanSwapper/2(MaxImag) -> Delay2/1
  Delay2/1 -> Slice3/1, Mult3/1, MaxImagOut/1, Phase_Detect/2
  Delay1/1 -> Phase_Detect/3, Mult2/1, MaxRealOut/1, Slice1/1
  Constant14/1 -> SwpRate/1
  SwpRate/1 -> LimitedAccum/4(SwpRate)
  [Locked] -> LimitedAccum/3(Locked)
  Gain_Master/1 -> GainOutMax/1, Mult3/2, Mult2/2  "GainMaster"
  Inverter2/1 -> Inverter/2
  Constant7/1 -> Gain/1
  Complex to Real-Imag2/2 -> Sign4/1
  Complex to Real-Imag2/1 -> Sign3/1
  Delay7/1 -> Complex to Real-Imag2/1
  Subtract1/1 -> Enabled Delay1/1
  Subtract/1 -> Enabled Delay/1
  Counter Limited/1 -> Delay8/1
  Enabled Delay/1 -> Abs/1
  Enabled Delay1/1 -> Abs1/1
  Mux/1 -> Scope3/1
  Mux13/1 -> Scope3/2
  Mux14/1 -> Scope3/3
  Sign2/1 -> Mux/1, Subtract/1
  Sign1/1 -> Subtract1/1, Mux13/1
  Sign3/1 -> Mux/2, Subtract/2
  Sign4/1 -> Mux13/2, Subtract1/2
  Delay8/1 -> Compare To Zero/1
  Abs/1 -> Add1/1, Mux14/1
  Abs1/1 -> Add1/2, Mux14/2
  Add1/1 -> Enabled Delay2/1, Display8/1, Scope3/4
  Enabled Delay2/1 -> Add1/3
  Compare To Zero/1 -> Enabled Delay2/2, Enabled Delay1/2, Enabled Delay/2
  GainOutMax/1 -> Display9/1
  GainOutMin/1 -> Display10/1
  [RawData] -> Delay7/1
  Manual Switch/1 -> ExtOffset Mixer1/1
  " Freq Offset Small"/1 -> Real-Imag to Complex3/2
  " Freq Offset Small"/2 -> Real-Imag to Complex3/1
  Real-Imag to Complex3/1 -> ExtOffset Mixer1/2
  Random Integer Generator1/1 -> Rate Transition1/1
  Rate Transition1/1 -> QPSK Modulator Baseband1/1
  QPSK Modulator Baseband1/1 -> Manual Switch/1
  BPSK Modulator Baseband/1 -> Manual Switch1/1
  FM Modulator Baseband/1 -> Manual Switch1/2
  Manual Switch1/1 -> Manual Switch/2

== system ComplexPhaseDetector/AD9957 ==
  In1 : Inport
  Add3 : Sum
  Complex to Real-Imag3 : ComplexToRealImag
  FIR Interpolation : dspmlti4/FIR Interpolation  FilterSource=Auto  h=designMultirateFIR(3,1)  L=8  FilterObject=FINTERP  framing=Allow multirate processing  outputBufInitCond=0  roundingMode=Floor  overflowMode=off  firstCoeffDataTypeStr=Inherit: Same word length as input  firstCoeffMin=[]  firstCoeffMax=[]  firstCoeffLastDataTypeStr=Inherit: Same word length as input  outputDataTypeStr=Inherit: Same as accumulator  outputMin=[]  outputMax=[]  outputLastDataTypeStr=Inherit: Same as accumulator
  NCO : dspsigops/NCO  AccIncSrc=Specify via dialog  AccInc=16384*3/8  PhaseOffsetSrc=Specify via dialog  PhaseOffset=0  AccumWL=16  HasDither=off  DitherWL=4  PNgeneratorLength=19  HasPhaseQuantizer=off  TableDepth=12  HasOutputPhaseError=off  Formula=Sine and cosine  DataType=double  OutputWL=16  OutputFL=14  CompMethod=Table lookup (no interpolation)  SampleTime=Ts/8  SamplesPerFrame=1  OutputFrames=off
  PhaseDetect1 : Product
  PhaseDetect2 : Product
  Out1 : Outport
  wires:
  In1/1 -> FIR Interpolation/1
  NCO/1 -> PhaseDetect2/2
  Complex to Real-Imag3/1 -> PhaseDetect1/1
  PhaseDetect2/1 -> Add3/1
  PhaseDetect1/1 -> Add3/2
  Complex to Real-Imag3/2 -> PhaseDetect2/1
  FIR Interpolation/1 -> Complex to Real-Imag3/1
  NCO/2 -> PhaseDetect1/2
  Add3/1 -> Out1/1

== system ComplexPhaseDetector/AD9957-2 ==
  In1 : Inport
  Add3 : Sum
  Complex to Real-Imag3 : ComplexToRealImag
  FIR Interpolation : dspmlti4/FIR Interpolation  FilterSource=Auto  h=designMultirateFIR(3,1)  L=8  FilterObject=FINTERP  framing=Allow multirate processing  outputBufInitCond=0  roundingMode=Floor  overflowMode=off  firstCoeffDataTypeStr=Inherit: Same word length as input  firstCoeffMin=[]  firstCoeffMax=[]  firstCoeffLastDataTypeStr=Inherit: Same word length as input  outputDataTypeStr=Inherit: Same as accumulator  outputMin=[]  outputMax=[]  outputLastDataTypeStr=Inherit: Same as accumulator
  NCO : dspsigops/NCO  AccIncSrc=Specify via dialog  AccInc=16384*3/8  PhaseOffsetSrc=Specify via dialog  PhaseOffset=0  AccumWL=16  HasDither=off  DitherWL=4  PNgeneratorLength=19  HasPhaseQuantizer=off  TableDepth=12  HasOutputPhaseError=off  Formula=Sine and cosine  DataType=double  OutputWL=16  OutputFL=14  CompMethod=Table lookup (no interpolation)  SampleTime=Ts/8  SamplesPerFrame=1  OutputFrames=off
  PhaseDetect1 : Product
  PhaseDetect2 : Product
  Out1 : Outport
  wires:
  Add3/1 -> Out1/1
  NCO/2 -> PhaseDetect1/2
  FIR Interpolation/1 -> Complex to Real-Imag3/1
  Complex to Real-Imag3/2 -> PhaseDetect2/1
  PhaseDetect1/1 -> Add3/2
  PhaseDetect2/1 -> Add3/1
  Complex to Real-Imag3/1 -> PhaseDetect1/1
  NCO/1 -> PhaseDetect2/2
  In1/1 -> FIR Interpolation/1

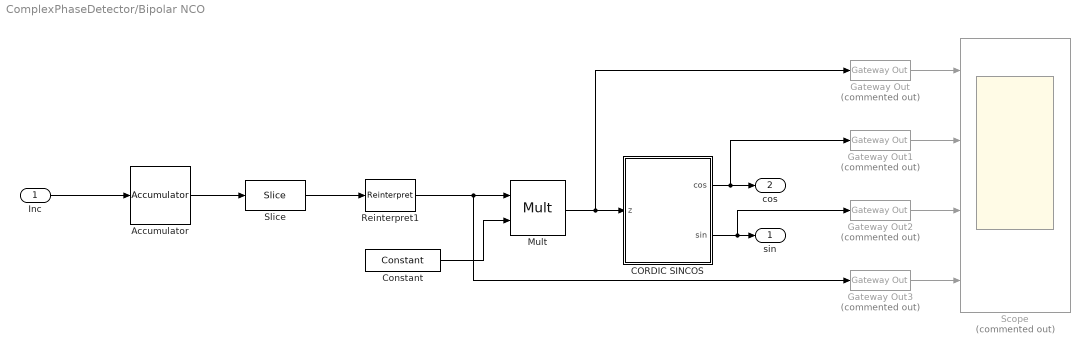
== system ComplexPhaseDetector/Bipolar NCO ==
  Inc : Inport
  Accumulator : xbsIndex_r4/Accumulator  operation=Add  n_bits=18+Bits  overflow=Wrap  scale=1  rst=off  hasbypass=off  infoeditControl=reset for floating point data type must be asserted for a minimum of 2 cycles  en=off  latency=1  msb_inp=100  msb=100  lsb=-100  use_behavioral_HDL=on  implementation=Fabric  dbl_ovrd=off  block_type=accum
  CORDIC SINCOS : Subsystem  mask(Xilinx CORDIC SINCOS){stages=17, pe_nbits=21, pe_binpt=17, pipeline_x=ones(1,17), prev_stages=17, pipeline=[1  1  1  1  1  1  1  1  1  1  1  1  1  1  1  1  1]}
      mask prompts: stages "Number of Processing Elements (integer value starting from 1)"; pe_nbits "Input Data Width"; pe_binpt "Input Binary Point Position"; pipeline_x "Latency for each Processing Element [1 0 0 1]"; prev_stages "Previous Number of Stages"; pipeline "Previous Pipeline Values"
      mask help: A parallel implementation, circular rotation mode CORDIC processor for calculating Sine and Cosine of input angle z. The number of iteration stages (and resultant output accuracy) and the processor arithmetic precision are controlled by the mask customization.
      mask init:
      | [bg,fg] = xlcmap('XBlock',0);
      | iPos = get_param(gcb,'Position');
      | iWidth=iPos(3)-iPos(1); iHeight=iPos(4)-iPos(2);
      | iCx=iWidth/2;
      | iCy=iHeight/2;
      | [logoX, logoY] = xlogo(iPos);
      | sav_gcb=gcb;
      | stages = round(sum(abs(stages)));
      | if (stages == 0)
      | 	stages = prev_stages;
      | end
      | x = zeros(1,stages);
      | pipe_size = max(size(pipeline_x));
      | if pipe_size >= stages
      | 	x(1,1:stages) = pipeline_x(1,1:stages);
      | else
      | 	x(1,1:pipe_size) = pipeline_x(1,1:pipe_size);
      | end
      | 
      | if (stages ~=prev_stages)
      | 	pipeline=x;
      | 	cordic_pe = find_system(gcb, 'lookUnderMasks', 'all', 'FollowLinks','on','masktype', 'CORDIC parallel PE');
      |     
      |   a=find_system(cordic_pe{1}, 'lookUnderMasks', 'all', 'FollowLinks','on','masktype', 'CORDIC iteration PE');
      |   for i= 2:length(a)
      |     for j=1:3
      | 	  delete_line(cordic_pe{1}, ['CORDIC PE' int2str(i-1) '/' int2str(j)], ['CORDIC PE' int2str(i) '/' int2str(j)]);
      |     end
      |   end
      |     if length(a)>0,
      |       delete_line(cordic_pe{1}, 'x/1', 'CORDIC PE1/1');
      |       delete_line(cordic_pe{1}, 'y/1', 'CORDIC PE1/2');
      |       delete_line(cordic_pe{1}, 'z/1', 'CORDIC PE1/3');
      |       delete_line(cordic_pe{1}, ['CORDIC PE' int2str(length(a)) '/1'],'X/1');
      |       delete_line(cordic_pe{1}, ['CORDIC PE' int2str(length(a)) '/2'],'Y/1');
      |       delete_line(cordic_pe{1}, ['CORDIC PE' int2str(length(a)) '/3'],'Terminator/1');
      |     elseif length(a)==0
      |       temp_port=get_param([cordic_pe{1} '/x'],'porthandles');
      |       temp_line=get_param(temp_port.Outport,'line');
      |       if temp_line>=0  delete_line(temp_line); end
      |       temp_port=get_param([cordic_pe{1} '/y'],'porthandles');
      |       temp_line=get_param(temp_port.Outport,'line');
      |       if temp_line>=0  delete_line(temp_line); end
      |       temp_port=get_param([cordic_pe{1} '/z'],'porthandles');
      |       temp_line=get_param(temp_port.Outport,'line');
      |       if temp_line>=0  delete_line(temp_line); end
      |     end
      | 
      |     for i=2:length(a)
      |       delete_block(a{i});
      |     end
      |     for i=2:stages,
      |         add_block([cordic_pe{1} '/CORDIC PE1'], [cordic_pe{1} '/CORDIC PE' int2str(i)], 'ii', int2str(i-1),'pe_nbits', 'pe_nbits','pe_binpt', 'pe_binpt','pipeline',['pipeline(1,' int2str(i) ')'],'position',[150+(i-1)*125, 70, 205+(i-1)*125, 130]);
      |     end
      | 
      |     for i= 2:stages,
      |       for j=1:3
      | 		add_line(cordic_pe{1}, ['CORDIC PE' int2str(i-1) '/' int2str(j)], ['CORDIC PE' int2str(i) '/' int2str(j)], 'autorouting', 'on');
      |       end
      |     end
      | 
      |     if stages==0
      |       add_line(cordic_pe{1}, 'x/1', 'X/1', 'autorouting', 'on');
      |       add_line(cordic_pe{1}, 'y/1', 'Terminator/1', 'autorouting', 'on');
      |       add_line(cordic_pe{1}, 'z/1', 'Z/1', 'autorouting', 'on');
      |     elseif stages>0
      |       add_line(cordic_pe{1}, 'x/1', 'CORDIC PE1/1', 'autorouting', 'on');
      |       add_line(cordic_pe{1}, 'y/1', 'CORDIC PE1/2', 'autorouting', 'on');
      |       add_line(cordic_pe{1}, 'z/1', 'CORDIC PE1/3', 'autorouting', 'on');
      | 
      |       set_param([cordic_pe{1} '/' 'X'], 'Position', [150+stages*125, 72, 180+stages*125, 86]);
      |       set_param([cordic_pe{1} '/' 'Y'], 'Position', [210+stages*125, 92, 225+stages*125, 108]);
      |       set_param([cordic_pe{1} '/' 'Terminator'], 'Position', [240+stages*125, 113, 270+stages*125, 127]);
      | 
      |       add_line(cordic_pe{1}, ['CORDIC PE' int2str(stages) '/1'], 'X/1', 'autorouting', 'on');
      |       add_line(cordic_pe{1}, ['CORDIC PE' int2str(stages) '/2'], 'Y/1', 'autorouting', 'on');
      |       add_line(cordic_pe{1}, ['CORDIC PE' int2str(stages) '/3'],'Terminator/1', 'autorouting', 'on');
      | 
      |       % force a "compile" of the constituent constant blocks to
      |       % workaround a data propagation problem
      |       find_system(cordic_pe{1}, 'lookUnderMasks', 'all', 'FollowLinks', 'on', 'MaskType','Xilinx Constant Block');
      |   end
      | 	set_param(sav_gcb, 'prev_stages', int2str(stages));
      | 	set_param(sav_gcb, 'pipeline', [ '[' int2str(x) ']']);
      | else
      | 	if (sum(pipeline~=x))
      | 		set_param(gcb, 'pipeline', [ '[' int2str(x) ']']);
      | 	end
      | end
      | str = sprintf('-%d',sum(x) + 3);
      settings: CopyFcn=set_param(gcb, 'MaskSelfModifiable', 'on', 'LinkStatus', 'none');
      mask Help: eval('');xlDoc('-book','sysgen','-topic','CORDIC_SINCOS');
      mask Display:
      | patch([0 iWidth iWidth 0],[0 0 iHeight iHeight] , bg);
      | patch(logoX,logoY , fg);
      | text(iCx-6,iCy,'z');
      | text(iCx,iCy+4,str);
      | port_label('input',1,'z');
      | port_label('output',1,'cos');
      | port_label('output',2,'sin');
      | plot([0 0 iWidth iWidth 0], [0 iHeight iHeight 0 0]);
  Constant : xbsIndex_r4/Constant  const=pi()  gui_display_data_type=Fixed-point  arith_type=Signed (2's comp)  n_bits=18  bin_pt=14  preci_type=Single  exp_width=8  frac_width=24  explicit_period=off  period=1  equ=P=C  opselect=C  inp2=PCIN>>17  opr=+  inp1=P  carry=CIN  dbl_ovrd=off  block_type=constant
  Gateway Out{,1..3} (4 alike) : xbsIndex_r4/Gateway Out  Commented=on  inherit_from_input=off  hdl_port=on  rows=1  columns=1  UseAsDAC=off  DACChannel='1'  interface=None  automatic_assignment=on  address_offset=hex2dec('00')  intf_name=''  intf_description=''  timing_constraint=None  locs_specified=off  LOCs={}  io_standard={}  block_type=gatewayout
  Mult : xbsIndex_r4/Mult  precision=User Defined  arith_type="Signed  (2's comp)"  n_bits=21  bin_pt=17  quantization=Truncate  overflow=Saturate  en=off  latency=3  use_behavioral_HDL=off  opt=Speed  use_embedded=on  optimum_pipeline=off  pipeline=on  dbl_ovrd=off  use_rpm=on  placement_style=Triangular  block_type=mult
  Reinterpret1 : xbsIndex_r4/Reinterpret  force_arith_type=on  arith_type="Signed  (2's comp)"  force_bin_pt=on  bin_pt=17  block_type=reinterpret
  Scope : Scope  Commented=on  NumInputPorts=4
  Slice : xbsIndex_r4/Slice  nbits=18  boolean_output=off  mode=Upper Bit Location + Width  bit1=0  base1=MSB of Input  bit0=0  base0=LSB of Input  dbl_ovrd=off  block_type=slice
  sin : Outport
  cos : Outport  Port=2
  wires:
  Mult/1 -> Gateway Out/1, CORDIC SINCOS/1(z)
  CORDIC SINCOS/1(cos) -> Gateway Out1/1, cos/1
  CORDIC SINCOS/2(sin) -> Gateway Out2/1, sin/1
  Gateway Out2/1 -> Scope/3
  Gateway Out/1 -> Scope/1
  Gateway Out1/1 -> Scope/2
  Accumulator/1 -> Slice/1
  Constant/1 -> Mult/2
  Gateway Out3/1 -> Scope/4
  Inc/1 -> Accumulator/1
  Slice/1 -> Reinterpret1/1
  Reinterpret1/1 -> Gateway Out3/1, Mult/1
